simulink model "ControlPenduloInvertidoLineal"  (R2024b)
settings: Solver=VariableStepAuto  StartTime=0.0  StopTime=50  RelTol=1e-3
libraries: fuzblock x1
settings Model: Creator=user  LastModifiedBy=user

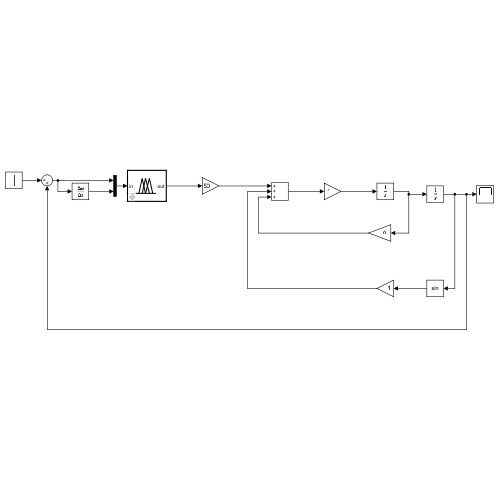
[thumbnail: Simulink's stored preview of the top-level diagram]
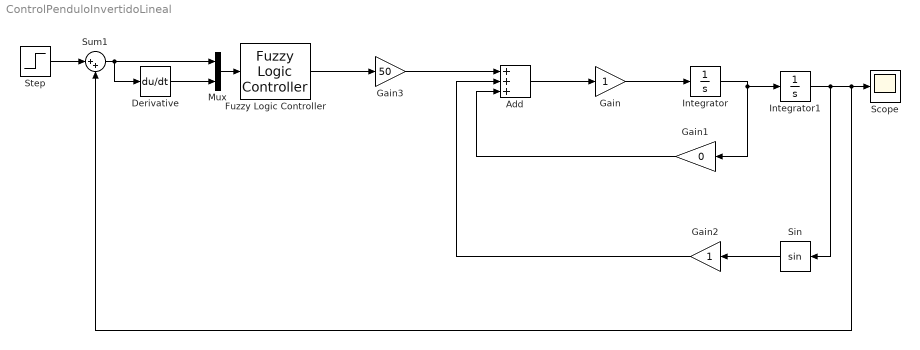
== system ControlPenduloInvertidoLineal ==
  Add : Sum  Inputs=+++
  Derivative : Derivative
  Fuzzy Logic Controller : fuzblock/Fuzzy Logic  Controller  FIS='tipper.fis'  OutputSampleNumber=101  DataType=double  FuzzifiedInputs=off  RuleFiringStrengths=off  RuleOutputs=off  AggregatedOutputs=off  SimulateUsing=Interpreted execution  OutOfRangeInputValueMessage=warning  NoRuleFiredMessage=warning  EmptyOutputFuzzySetMessage=warning
  Gain : Gain
  Gain1 : Gain  Gain=0
  Gain2 : Gain
  Gain3 : Gain  Gain=50
  Integrator : Integrator
  Integrator1 : Integrator  InitialCondition=0.1
  Mux : Mux  Inputs=2
  Scope : Scope
  Sin : Trigonometry
  Step : Step  SampleTime=0
  Sum1 : Sum  Inputs=|++
  wires:
  Add/1 -> Gain/1
  Gain/1 -> Integrator/1
  Integrator/1 -> Gain1/1, Integrator1/1
  Gain1/1 -> Add/3
  Gain2/1 -> Add/2
  Sin/1 -> Gain2/1
  Step/1 -> Sum1/1
  Derivative/1 -> Mux/2
  Sum1/1 -> Derivative/1, Mux/1
  Mux/1 -> Fuzzy Logic Controller/1
  Gain3/1 -> Add/1
  Fuzzy Logic Controller/1 -> Gain3/1
  Integrator1/1 -> Sin/1, Sum1/2, Scope/1
